simulink model "danxiangbanboqiaoshizhengliu_m2"  (Simulink 8.5)
settings: Solver=ode15s  StartTime=0.0  StopTime=0.2  RelTol=1e-3
libraries: powerlib x10
settings Model: Creator=Administrator  LastModifiedBy=佳君
settings DebuggingCC: SolverPrmCheckMsg=warning  FcnCallInpInsideContextMsg=UseLocalSettings  StrictBusMsg=Warning

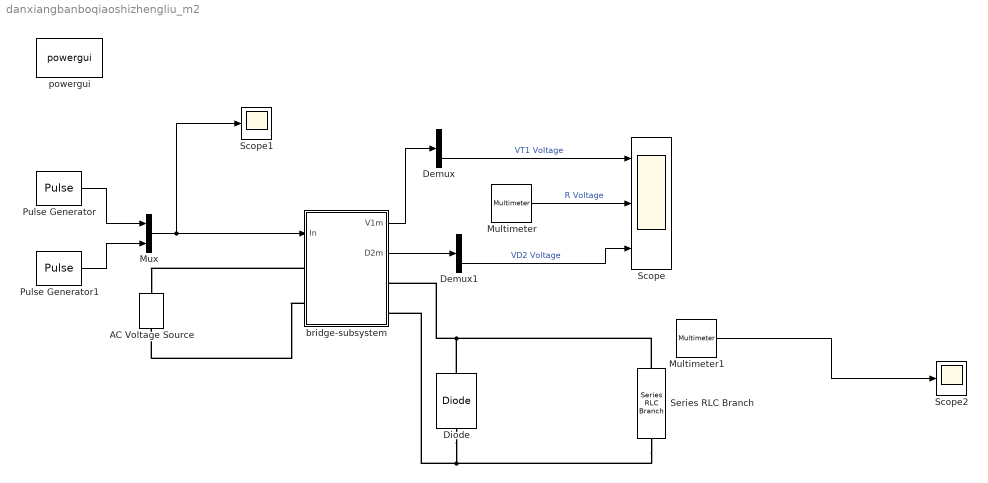
== system danxiangbanboqiaoshizhengliu_m2 ==
  AC Voltage Source : powerlib/Electrical Sources/AC Voltage Source  Amplitude=220  Phase=0  Frequency=50  SampleTime=0  Measurements=Voltage
  Demux : Demux  Outputs=2
  Demux1 : Demux  Outputs=2
  Diode : powerlib/Power Electronics/Diode  Ron=0.001  Lon=0  Vf=0.8  IC=0  UseSnubber=off  Rs=500  Cs=250e-9  Measurements=off
  Multimeter : powerlib/Measurements/Multimeter  PhasorSimulation=off  OutputType=Complex  sel=1  L=3  Gain=1  yselected={'Ub: Series RLC Branch'};  PSBOutputType=1  PSBequivalent=0  AxesSetting=[0,0.1,-100,100]  Display=0  SavedBlockNames=-11
  Multimeter1 : powerlib/Measurements/Multimeter  PhasorSimulation=off  OutputType=Complex  sel=3  L=3  Gain=1  yselected={'Ib: Series RLC Branch'};  PSBOutputType=1  PSBequivalent=0  AxesSetting=[0,0.1,-100,100]  Display=0  SavedBlockNames=-11
  Mux : Mux  Inputs=2
  Pulse Generator : DiscretePulseGenerator  PulseType=Time based  Period=1/50  PulseWidth=5  PhaseDelay=0.00167
  Pulse Generator1 : DiscretePulseGenerator  PulseType=Time based  Period=1/50  PulseWidth=5  PhaseDelay=0.00167*7
  Scope : Scope  NumInputPorts=3
      settings: YMin=0~-2.5~-0.25  YMax=60000~42.5~3.5
  Scope1 : Scope
  Scope2 : Scope
      settings: YMin=-0.1  YMax=2.2  SaveName=ScopeData2
  Series RLC Branch : powerlib/Elements/Series RLC Branch  LConnTagsString=__new0  RConnTagsString=__new0  BranchType=L  Resistance=10  Inductance=11  SetiL0=off  InitialCurrent=0  Capacitance=1e-6  Setx0=off  InitialVoltage=0  Measurements=Branch voltage and current
  bridge-subsystem : Subsystem
  powergui : powerlib/powergui  Priority=1  SimulationMode=Continuous  SolverType=Tustin/Backward Euler (TBE)  SampleTime=50e-6  frequency=60  SPID=off  DisableSnubberDevices=off  DisableRonSwitches=off  DisableVfSwitches=off  SwTol=0  DisplayEquations=off  Interpol=off  methode=off  Ts=0  FunctionMessages=off  echomessages=off  HookPort=off  EnableUseOfTLC=off  x0status=blocks  frequencyindice=50  Pbase=100e6  ErrMax=1e-4  Iterations=50  UnitsV=kV  UnitsW=MW  buscounter=0  RestoreLinks=warning  ResistiveCurrentMeasurement=off  Frange=[0:2:500]  Ylog=off  Xlog=on  ShowGrid=off  save=off  variable=ZData  structure=0  ZoomFFT=on  StartTime=0.0  cycles=1  DisplayStyle=1  fundamental=60  FreqAxis=off  MaxFrequency=1000  frequencyindicesteady=1  RmsSteady=1  display=off
  wires:
  Pulse Generator/1 -> Mux/1
  Pulse Generator1/1 -> Mux/2
  bridge-subsystem/1(V1m) -> Demux/1
  Mux/1 -> Scope1/1, bridge-subsystem/1(In)
  bridge-subsystem/2(D2m) -> Demux1/1
  Multimeter/1 -> Scope/2  "R Voltage"
  Demux1/2 -> Scope/3  "VD2 Voltage"
  Demux/2 -> Scope/1  "VT1 Voltage"
  Multimeter1/1 -> Scope2/1
  connections:
  Series RLC Branch/LConn1 -- Diode/RConn1 -- bridge-subsystem/RConn1
  Series RLC Branch/RConn1 -- Diode/LConn1 -- bridge-subsystem/RConn2
  bridge-subsystem/LConn2 -- AC Voltage Source/LConn1
  bridge-subsystem/LConn1 -- AC Voltage Source/RConn1

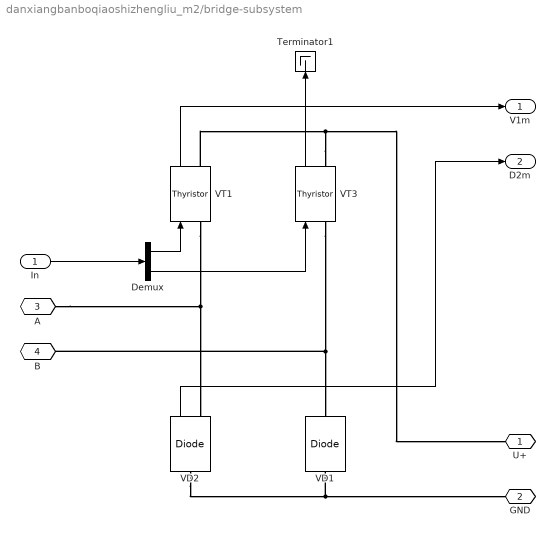
== system danxiangbanboqiaoshizhengliu_m2/bridge-subsystem ==
  In : Inport
  Demux : Demux  Outputs=2
  Terminator1 : Terminator
  VD1 : powerlib/Power Electronics/Diode  Ron=0.001  Lon=0  Vf=0.8  IC=0  UseSnubber=off  Rs=500  Cs=250e-9  Measurements=off
  VD2 : powerlib/Power Electronics/Diode  Ron=0.001  Lon=0  Vf=0.8  IC=0  UseSnubber=off  Rs=500  Cs=250e-9  Measurements=on
  VT1 : powerlib/Power Electronics/Thyristor  Ron=0.001  Lon=0  Vf=0.8  IC=0  Rs=500  Cs=250e-9  Measurements=on
  VT3 : powerlib/Power Electronics/Thyristor  Ron=0.001  Lon=0  Vf=0.8  IC=0  Rs=500  Cs=250e-9  Measurements=on
  "U+ " : PMIOPort  Port=1  Side=Right
  GND : PMIOPort  Port=2  Side=Right
  A : PMIOPort  Port=3  Side=Left
  B : PMIOPort  Port=4  Side=Left
  V1m : Outport
  D2m : Outport  Port=2
  wires:
  In/1 -> Demux/1
  VT3/1 -> Terminator1/1
  VD2/1 -> D2m/1
  Demux/1 -> VT1/1
  Demux/2 -> VT3/1
  VT1/1 -> V1m/1
  connections:
  VT3/RConn1 -- "U+ "/RConn1 -- VT1/RConn1
  VT3/LConn1 -- VD1/RConn1 -- B/RConn1
  VT1/LConn1 -- VD2/RConn1 -- A/RConn1
  VD1/LConn1 -- GND/RConn1 -- VD2/LConn1
